simulink model "ACE_II_AC_DCMotor"  (R2025b)
settings: Solver=FixedStepAuto  StartTime=0.0  StopTime=10.0  FixedStep=T  MaxStep=0.2  RelTol=1e-3
undefined symbols (not defined in the file): b, J, Km, q0, q1, T
libraries: simulink x1
settings Model: Creator=Felix  LastModifiedBy=Felix

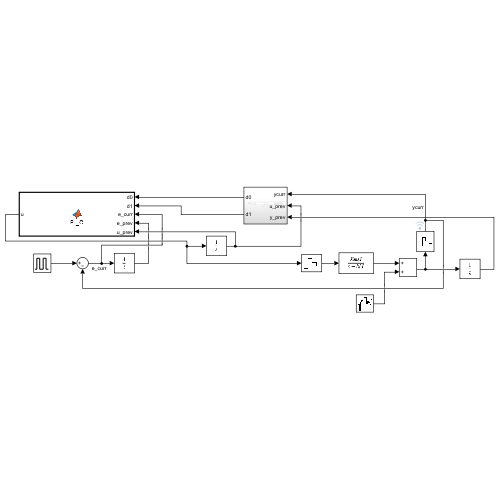
[thumbnail: Simulink's stored preview of the top-level diagram]
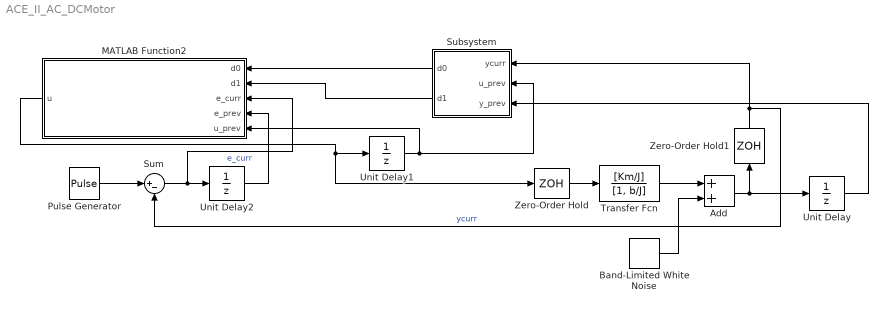
== system ACE_II_AC_DCMotor ==
  Add : Sum
  Band-Limited White Noise : simulink/Sources/Band-Limited White Noise  Cov=[0.001]  Ts=T  seed=[23341]
  MATLAB Function2 : MATLAB Function  TreatAsAtomicUnit=on
  Pulse Generator : DiscretePulseGenerator  PulseType=Time based  Amplitude=50  Period=4  PulseWidth=50
  Subsystem : Subsystem
  Sum : Sum  Inputs=|+-
  Transfer Fcn : TransferFcn  Numerator=[Km/J]  Denominator=[1, b/J]
  Unit Delay : UnitDelay  SampleTime=-1  HasFrameUpgradeWarning=on
  Unit Delay1 : UnitDelay  SampleTime=-1  HasFrameUpgradeWarning=on
  Unit Delay2 : UnitDelay  SampleTime=-1  HasFrameUpgradeWarning=on
  Zero-Order Hold : ZeroOrderHold  SampleTime=-1
  Zero-Order Hold1 : ZeroOrderHold  SampleTime=-1
  wires:
  Zero-Order Hold/1 -> Transfer Fcn/1
  Transfer Fcn/1 -> Add/1
  Band-Limited White Noise/1 -> Add/2
  Add/1 -> Zero-Order Hold1/1, Unit Delay/1
  MATLAB Function2/1(u) -> Zero-Order Hold/1, Unit Delay1/1
  Zero-Order Hold1/1 -> Subsystem/1(ycurr), Sum/2  "ycurr"
  Pulse Generator/1 -> Sum/1
  Sum/1 -> Unit Delay2/1, MATLAB Function2/3(e_curr)  "e_curr"
  Unit Delay2/1 -> MATLAB Function2/4(e_prev)
  Unit Delay1/1 -> Subsystem/2(u_prev), MATLAB Function2/5(u_prev)
  Unit Delay/1 -> Subsystem/3(y_prev)
  Subsystem/1(d0) -> MATLAB Function2/1(d0)
  Subsystem/2(d1) -> MATLAB Function2/2(d1)

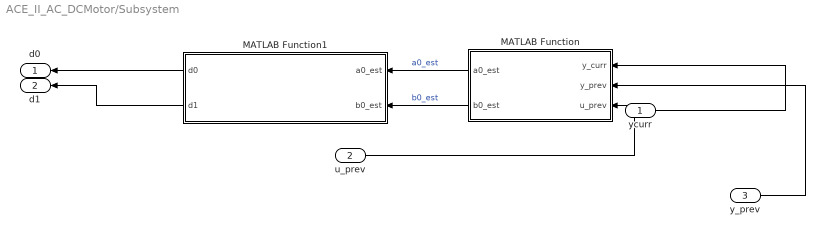
== system ACE_II_AC_DCMotor/Subsystem ==
  ycurr : Inport
  u_prev : Inport  Port=2
  y_prev : Inport  Port=3
  MATLAB Function : MATLAB Function  TreatAsAtomicUnit=on
  MATLAB Function1 : MATLAB Function  TreatAsAtomicUnit=on
  d0 : Outport
  d1 : Outport  Port=2
  wires:
  MATLAB Function/2(b0_est) -> MATLAB Function1/2(b0_est)  "b0_est"
  y_prev/1 -> MATLAB Function/2(y_prev)
  MATLAB Function/1(a0_est) -> MATLAB Function1/1(a0_est)  "a0_est"
  MATLAB Function1/2(d1) -> d1/1
  ycurr/1 -> MATLAB Function/1(y_curr)
  u_prev/1 -> MATLAB Function/3(u_prev)
  MATLAB Function1/1(d0) -> d0/1

== matlab function ACE_II_AC_DCMotor/Subsystem/MATLAB Function1 ==
  data: a0_est input; b0_est input; q0 parameter; q1 parameter; d0 output; d1 output
function [d0,d1] =pole_placement_controller(a0_est,b0_est,q0,q1)

d0 = (q0 + a0_est) / b0_est;
d1 = (q1 + 1 - a0_est) / b0_est;

== matlab function ACE_II_AC_DCMotor/Subsystem/MATLAB Function ==
  data: y_curr input; y_prev input; a0_est output; u_prev input; b0_est output
function [a0_est, b0_est] = rls_estimator(y_curr, y_prev, u_prev)
    % 1. DEFINE PERSISTENT VARIABLES
    % These act like global variables in an Arduino loop. 
    % They remember their values from the previous time step.
    persistent P xe initialized
    
    % 2. INITIALIZATION (Runs only once at the very beginning)
    if isempty(initialized)
        P = 100 * eye(2);       % Initial Covariance matrix
        xe = [-0.5; 1.0];       % Initial guess for [a0; b0]
        initialized = true;
    end
    
    alpha = 1.0; % Forgetting factor (1.0 = remember everything)
    
    % 3. RECURSIVE LEAST SQUARES MATH
    % The measurement vector based on past inputs/outputs
    C = [-y_prev, u_prev];
    
    % Calculate the Kalman Gain (L)
    % We use scalar division '/' here to avoid the singular matrix error
    denominator = (C * P * C') + alpha;
    L = (P * C') / denominator;
    
    % Calculate the error between the actual motor speed and our prediction
    y_prediction = C * xe;
    error = y_curr - y_prediction;
    
    % Update the parameter estimates based on the error
    xe = xe + L * error;
    
    % Update the Covariance matrix for the next step
    P = (eye(2) - L * C) * P / alpha;
    
    % 4. ASSIGN OUTPUTS
    a0_est = xe(1);
    b0_est = xe(2);
end

== matlab function ACE_II_AC_DCMotor/MATLAB Function2 ==
  data: d0 input; d1 input; u output; e_curr input; e_prev input; u_prev input
function u = PI_C(d0,d1, e_curr, e_prev, u_prev)
u= u_prev + (d1 * e_curr) + (d0 * e_prev);
